simulink model "TrajectoryTracking_2015b_000"  (R2017a)
settings: Solver=ode45  StartTime=0.0  StopTime=125  RelTol=1e-3
values from neighbouring files (symbols this model uses):
  tau_d_1 = C_RB1+C_A1+D1+G1    [DesiredInputOptimalConfiguration.m]
  tau_d_2 = C_RB2+C_A2+D2+G2    [DesiredInputOptimalConfiguration.m]
  tau_d_3 = C_RB3+C_A3+D3+G3    [DesiredInputOptimalConfiguration.m]
  tau_d_4 = C_RB4+C_A4+D4+G4    [DesiredInputOptimalConfiguration.m]
  tau_d_5 = C_RB5+C_A5+D5+G5    [DesiredInputOptimalConfiguration.m]
  tau_d_6 = C_RB6+C_A6+D6+G6    [DesiredInputOptimalConfiguration.m]
  tau_d_7 = C_RB7+C_A7+D7+G7    [DesiredInputOptimalConfiguration.m]
undefined symbols (not defined in the file or in its folder): angular_velocity_pitch_1, angular_velocity_pitch_2, angular_velocity_roll_1, angular_velocity_roll_2, angular_velocity_yaw_1, angular_velocity_yaw_2, B_input, d_H, K1, K2, linear_velocity_x_1, linear_velocity_x_2, linear_velocity_y_1, linear_velocity_y_2, linear_velocity_z_1, linear_velocity_z_2, pitch_angle_1, pitch_angle_2, roll_angle_1, roll_angle_2, t_1_last, t_e_1, t_e_2, u_d_1, u_d_2, u_d_optimized, veh, x1, x2, y1, y2, yaw_angle_1, yaw_angle_2, z1, z2
undefined symbols (not defined in the file): a_F1, a_F2, a_F3, a_F4, b_F1, b_F2, b_F3, b_F4, b_T1_optimized, b_T2_optimized, d_T1_optimized, d_T2_optimized, gamma_F1_optimized, gamma_F2_optimized, gamma_F3_optimized, gamma_F4_optimized, r_T1_optimized, r_T2_optimized, x_F1_optimized, x_F2_optimized, x_F3_optimized, x_F4_optimized
libraries: sharedtransform x1, shared6dofsys x1
(part 1 of 2)
settings Model: Creator=yongyu  LastModifiedBy=yongyu
settings OptimizationCC: LifeSpan=inf
settings DebuggingCC: SFExecutionAtInitializationDiag=none
settings HardwareCC: ProdBitPerSizeT=32  ProdBitPerPtrDiffT=32  ProdWordSize=32  ProdHWDeviceType=Specified

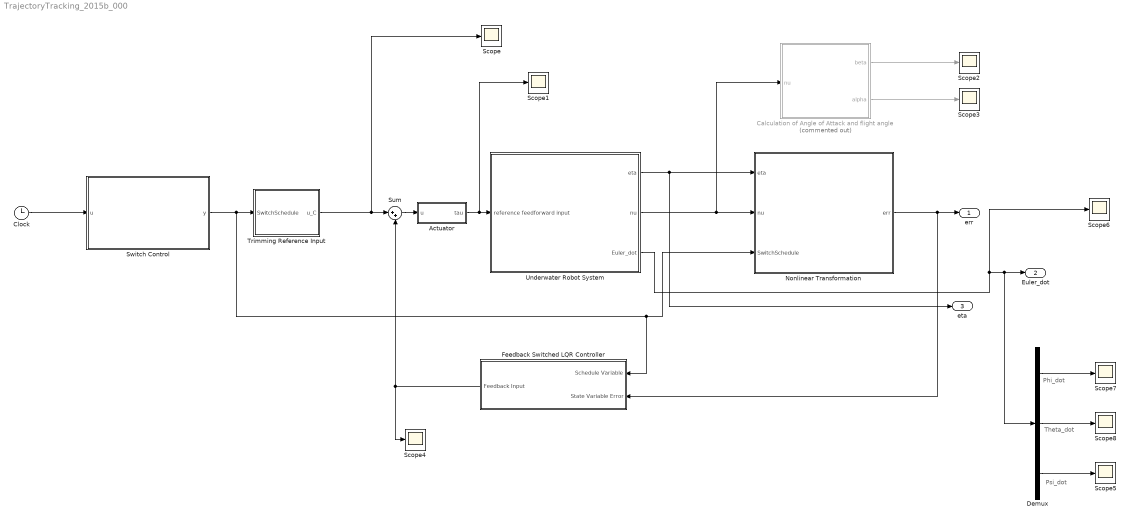
== system TrajectoryTracking_2015b_000 ==
  note: Theta_dot
  note: Phi_dot
  note: Psi_dot
  Actuator : Subsystem
  Calculation of Angle of Attack and flight angle : Subsystem  Commented=on
  Clock : Clock
  Demux : Demux  Outputs=3
  Feedback Switched LQR Controller : Subsystem
  Nonlinear Transformation : Subsystem
  Scope{,1..8} (9 alike) : Scope
  Sum : Sum  Inputs=|++
  Switch Control : MATLAB Function  TreatAsAtomicUnit=on
  "Trimming Reference Input " : Subsystem
  Underwater Robot System : Subsystem
  err : Outport
  Euler_dot : Outport  Port=2
  eta : Outport  Port=3
  wires:
  Nonlinear Transformation/1(err) -> err/1, Feedback Switched LQR Controller/2(State Variable Error)
  Calculation of Angle of Attack and flight angle/2(alpha) -> Scope3/1
  Calculation of Angle of Attack and flight angle/1(beta) -> Scope2/1
  "Trimming Reference Input "/1(u_C) -> Scope/1, Sum/1
  Underwater Robot System/1(eta) -> eta/1, Nonlinear Transformation/1(eta)
  Underwater Robot System/2(nu) -> Calculation of Angle of Attack and flight angle/1(nu), Nonlinear Transformation/2(nu)
  Underwater Robot System/3(Euler_dot) -> Scope6/1, Demux/1, Euler_dot/1
  Clock/1 -> Switch Control/1(u)
  Demux/3 -> Scope5/1
  Switch Control/1(y) -> Feedback Switched LQR Controller/1(Schedule Variable), Nonlinear Transformation/3(SwitchSchedule), "Trimming Reference Input "/1(SwitchSchedule)
  Demux/1 -> Scope7/1
  Demux/2 -> Scope8/1
  Sum/1 -> Actuator/1(u)
  Actuator/1(tau) -> Scope1/1, Underwater Robot System/1("reference feedforward input ")
  Feedback Switched LQR Controller/1(Feedback Input) -> Sum/2, Scope4/1

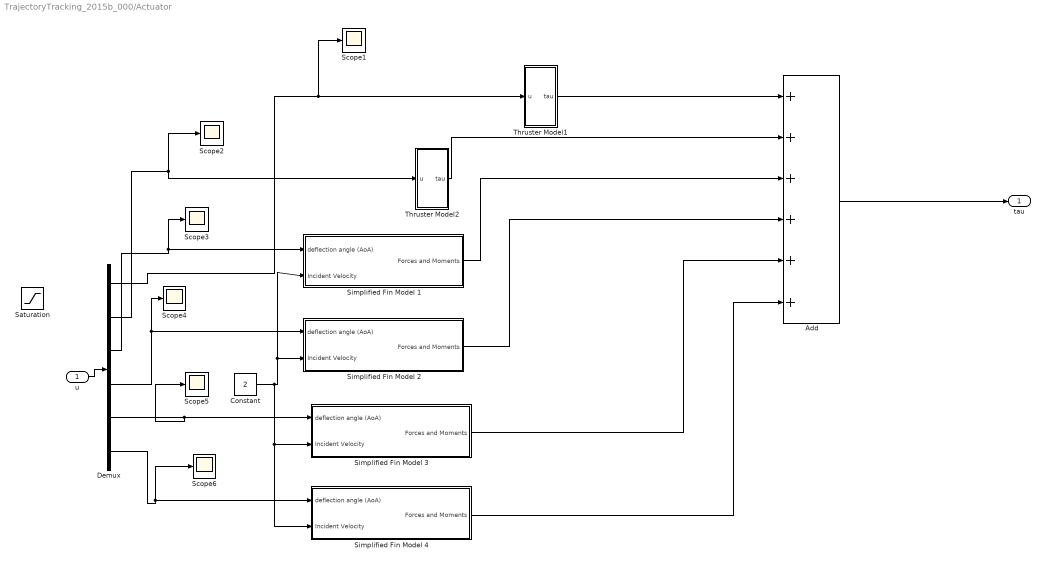
== system TrajectoryTracking_2015b_000/Actuator ==
  u : Inport
  Add : Sum  Inputs=++++++
  Constant : Constant  Value=2
  Demux : Demux  Outputs=6
  Saturation : Saturate  UpperLimit=[40 40 40 40 40 40]  LowerLimit=[-35 -35 -35 -35 -35 -35]
  Scope{1..6} (6 alike) : Scope
  "Simplified Fin Model 1 " : Subsystem  mask{x_F=x_F1_optimized, gama_F=gamma_F1_optimized, a_F=a_F1, b_F=b_F1, C_L=0.3, C_D=0, d_H=d_H, rho=1033}
      mask prompts: x_F "Position of fin middle in body frame {b} in cylinderic coordinate"; gama_F "Rotation angle of the fin (radian)"; a_F "Length of the fin (m)"; b_F "Width of the fin (m)"; C_L "Lift coefficient"; C_D "Drag coefficient"; d_H "Diameter of hull cylinder (m)"; rho "Fluid density"
      mask DialogControl DescTextVar Prompt: Simplified Model for fin (under assumption of small angle of attack)
  Simplified Fin Model 2 : Subsystem  mask{x_F=x_F2_optimized, gama_F=gamma_F2_optimized, a_F=a_F2, b_F=b_F2, C_L=0.3, C_D=0, d_H=d_H, rho=1033}
      mask prompts: x_F "Position of fin middle in body frame {b} in cylinderic coordinate"; gama_F "Rotation angle of the fin (radian)"; a_F "Length of the fin (m)"; b_F "Width of the fin (m)"; C_L "Lift coefficient"; C_D "Drag coefficient"; d_H "Diameter of hull cylinder (m)"; rho "Fluid density"
      mask DialogControl DescTextVar Prompt: Simplified Model for fin (under assumption of small angle of attack)
  Simplified Fin Model 3 : Subsystem  mask{x_F=x_F3_optimized, gama_F=gamma_F3_optimized, a_F=a_F3, b_F=b_F3, C_L=0.3, C_D=0, d_H=d_H, rho=1033}
      mask prompts: x_F "Position of fin middle in body frame {b} in cylinderic coordinate"; gama_F "Rotation angle of the fin (radian)"; a_F "Length of the fin (m)"; b_F "Width of the fin (m)"; C_L "Lift coefficient"; C_D "Drag coefficient"; d_H "Diameter of hull cylinder (m)"; rho "Fluid density"
      mask DialogControl DescTextVar Prompt: Simplified Model for fin (under assumption of small angle of attack)
  Simplified Fin Model 4 : Subsystem  mask{x_F=x_F4_optimized, gama_F=gamma_F4_optimized, a_F=a_F4, b_F=b_F4, C_L=0.3, C_D=0, d_H=d_H, rho=1033}
      mask prompts: x_F "Position of fin middle in body frame {b} in cylinderic coordinate"; gama_F "Rotation angle of the fin (radian)"; a_F "Length of the fin (m)"; b_F "Width of the fin (m)"; C_L "Lift coefficient"; C_D "Drag coefficient"; d_H "Diameter of hull cylinder (m)"; rho "Fluid density"
      mask DialogControl DescTextVar Prompt: Simplified Model for fin (under assumption of small angle of attack)
  Thruster Model1 : Subsystem  mask{d_T=d_T1_optimized, b_T=b_T1_optimized, r_T=r_T1_optimized, lambda_T=veh.lambda1}
      mask DialogControl DescTextVar Prompt: Model of Thruster
  Thruster Model2 : Subsystem  mask{d_T=d_T2_optimized, b_T=b_T2_optimized, r_T=r_T2_optimized, lambda_T=veh.lambda2}
      mask DialogControl DescTextVar Prompt: Model of Thruster
  tau : Outport
  wires:
  Simplified Fin Model 3/1(Forces and Moments) -> Add/5
  "Simplified Fin Model 1 "/1(Forces and Moments) -> Add/3
  Simplified Fin Model 2/1(Forces and Moments) -> Add/4
  Thruster Model2/1(tau) -> Add/2
  Simplified Fin Model 4/1(Forces and Moments) -> Add/6
  Add/1 -> tau/1
  Thruster Model1/1(tau) -> Add/1
  Demux/1 -> Thruster Model1/1(u), Scope1/1
  Demux/2 -> Thruster Model2/1(u), Scope2/1
  Demux/3 -> "Simplified Fin Model 1 "/1(deflection angle (AoA)), Scope3/1
  Demux/4 -> Scope4/1, Simplified Fin Model 2/1(deflection angle (AoA))
  Demux/5 -> Scope5/1, Simplified Fin Model 3/1(deflection angle (AoA))
  Demux/6 -> Simplified Fin Model 4/1(deflection angle (AoA)), Scope6/1
  u/1 -> Demux/1
  Constant/1 -> Simplified Fin Model 4/2(Incident Velocity), Simplified Fin Model 3/2(Incident Velocity), Simplified Fin Model 2/2(Incident Velocity), "Simplified Fin Model 1 "/2(Incident Velocity)

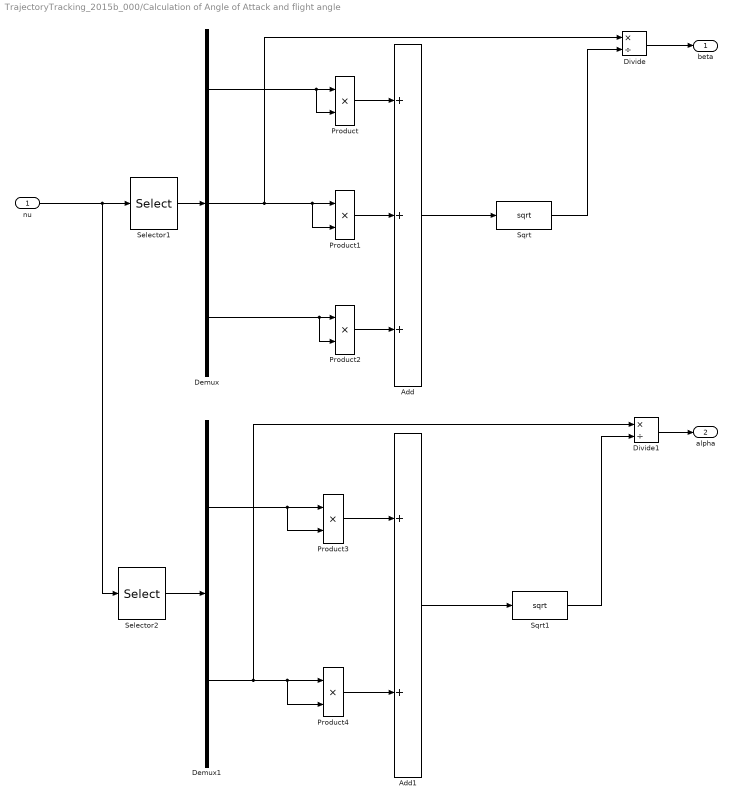
== system TrajectoryTracking_2015b_000/Calculation of Angle of Attack and flight angle ==
  nu : Inport
  Add : Sum  Inputs=+++
  Add1 : Sum
  Demux : Demux  Outputs=3
  Demux1 : Demux  Outputs=2
  Divide : Product  Inputs=*/
  Divide1 : Product  Inputs=*/
  Product{,1..4} (5 alike) : Product
  Selector1 : Selector  InputPortWidth=6  IndexOptions=Index vector (dialog)  Indices=[1 2 3]  OutputSizes=1
  Selector2 : Selector  InputPortWidth=6  IndexOptions=Index vector (dialog)  Indices=[1 3]  OutputSizes=1
  Sqrt : Sqrt  SaturateOnIntegerOverflow=on
  Sqrt1 : Sqrt  SaturateOnIntegerOverflow=on
  beta : Outport
  alpha : Outport  Port=2
  wires:
  nu/1 -> Selector2/1, Selector1/1
  Selector1/1 -> Demux/1
  Demux/1 -> Product/2, Product/1
  Demux/2 -> Product1/2, Product1/1, Divide/1
  Demux/3 -> Product2/2, Product2/1
  Product/1 -> Add/1
  Product1/1 -> Add/2
  Product2/1 -> Add/3
  Add/1 -> Sqrt/1
  Sqrt/1 -> Divide/2
  Divide/1 -> beta/1
  Selector2/1 -> Demux1/1
  Demux1/1 -> Product3/2, Product3/1
  Demux1/2 -> Divide1/1, Product4/2, Product4/1
  Product3/1 -> Add1/1
  Product4/1 -> Add1/2
  Add1/1 -> Sqrt1/1
  Sqrt1/1 -> Divide1/2
  Divide1/1 -> alpha/1

== system TrajectoryTracking_2015b_000/Feedback Switched LQR Controller ==
  Schedule Variable : Inport
  State Variable Error : Inport  Port=2
  Constant1 : Constant  Value=-K2
  Constant7 : Constant  Value=-K1
  Multiport Switch : MultiPortSwitch  Inputs=2
  Product : Product  Multiplication=Matrix(*)
  Feedback Input : Outport
  wires:
  Constant7/1 -> Multiport Switch/2
  Constant1/1 -> Multiport Switch/3
  Multiport Switch/1 -> Product/1
  Product/1 -> Feedback Input/1
  State Variable Error/1 -> Product/2
  Schedule Variable/1 -> Multiport Switch/1

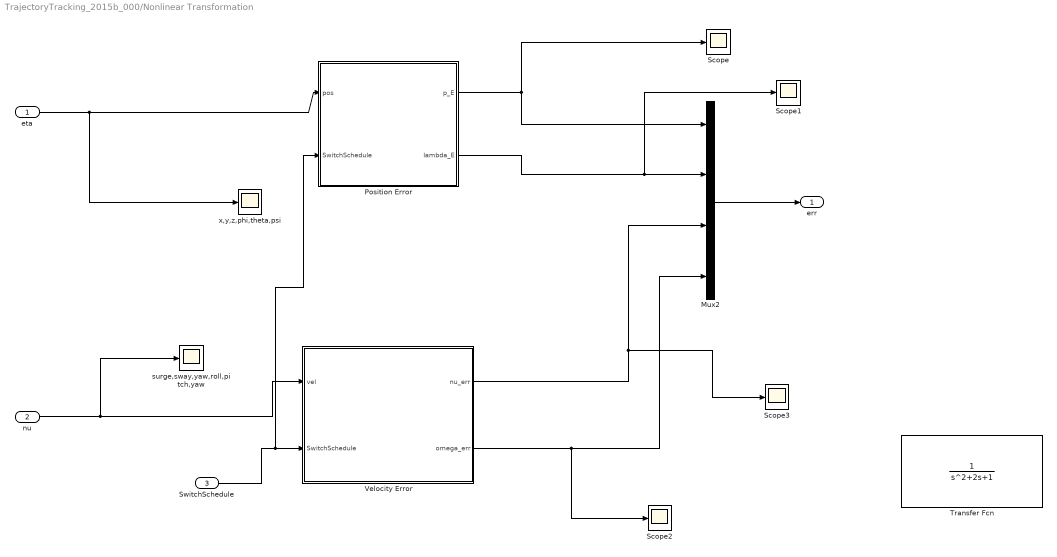
== system TrajectoryTracking_2015b_000/Nonlinear Transformation ==
  eta : Inport
  nu : Inport  Port=2
  SwitchSchedule : Inport  Port=3
  Mux2 : Mux
  "Position Error " : Subsystem
  Scope{,1..3} (4 alike) : Scope
  Transfer Fcn : TransferFcn
  "Velocity Error " : Subsystem
  surge,sway,yaw,roll,pitch,yaw : Scope
  x,y,z,phi,theta,psi : Scope
  err : Outport
  wires:
  nu/1 -> surge,sway,yaw,roll,pitch,yaw/1, "Velocity Error "/1(vel)
  eta/1 -> x,y,z,phi,theta,psi/1, "Position Error "/1(pos)
  Mux2/1 -> err/1
  "Position Error "/1(p_E) -> Scope/1, Mux2/1
  "Position Error "/2(lambda_E) -> Scope1/1, Mux2/2
  "Velocity Error "/1(nu_err) -> Scope3/1, Mux2/3
  "Velocity Error "/2(omega_err) -> Scope2/1, Mux2/4
  SwitchSchedule/1 -> "Position Error "/2(SwitchSchedule), "Velocity Error "/2(SwitchSchedule)

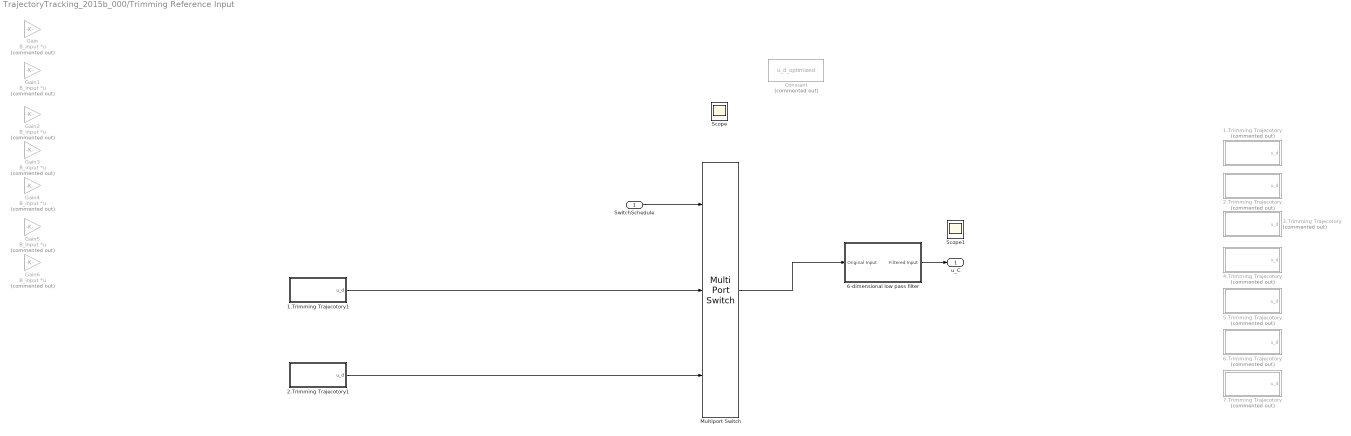
== system TrajectoryTracking_2015b_000/Trimming Reference Input  ==
  SwitchSchedule : Inport
  1.Trimming Trajecotory : Subsystem  Commented=on
  1.Trimming Trajecotory1 : Subsystem
  2.Trimming Trajecotory : Subsystem  Commented=on
  2.Trimming Trajecotory1 : Subsystem
  3.Trimming Trajecotory : Subsystem  Commented=on
  4.Trimming Trajecotory : Subsystem  Commented=on
  5.Trimming Trajecotory : Subsystem  Commented=on
  6-dimensional low pass filter : Subsystem
  6.Trimming Trajecotory : Subsystem  Commented=on
  7.Trimming Trajecotory : Subsystem  Commented=on
  Constant : Constant  Commented=on  Value=u_d_optimized
  Gain{,1..6} (7 alike) : Gain  Commented=on  Gain=B_input  Multiplication=Matrix(K*u)
  Multiport Switch : MultiPortSwitch  Inputs=2
  Scope : Scope
  Scope1 : Scope
  u_C : Outport
  wires:
  SwitchSchedule/1 -> Multiport Switch/1
  1.Trimming Trajecotory1/1(u_d) -> Multiport Switch/2
  6-dimensional low pass filter/1(Filtered Input) -> u_C/1
  Multiport Switch/1 -> 6-dimensional low pass filter/1(Original Input)
  2.Trimming Trajecotory1/1(u_d) -> Multiport Switch/3

== system TrajectoryTracking_2015b_000/Underwater Robot System ==
  "reference feedforward input " : Inport
  Demux : Demux  Outputs=6
  Underwater Robot System : Subsystem
  eta : Outport
  nu : Outport  Port=2
  Euler_dot : Outport  Port=3
  wires:
  Underwater Robot System/1(eta) -> eta/1
  Underwater Robot System/2(nu) -> nu/1
  Demux/6 -> Underwater Robot System/6(N)
  Demux/5 -> Underwater Robot System/5(M)
  Demux/4 -> Underwater Robot System/4(K)
  Demux/3 -> Underwater Robot System/3(Z)
  Demux/2 -> Underwater Robot System/2(Y)
  Demux/1 -> Underwater Robot System/1(X)
  "reference feedforward input "/1 -> Demux/1
  Underwater Robot System/3(Euler_dot) -> Euler_dot/1

== system TrajectoryTracking_2015b_000/Actuator/Simplified Fin Model 1  ==
  deflection angle (AoA) : Inport
  Incident Velocity : Inport  Port=2
  Drag Forces and Moments : Subsystem
  Lift Forces and Moments : Subsystem
  Sum : Sum  Inputs=|++
  Forces and Moments : Outport
  wires:
  deflection angle (AoA)/1 -> Drag Forces and Moments/1(AoA), Lift Forces and Moments/1(AoA)
  Incident Velocity/1 -> Drag Forces and Moments/2(u), Lift Forces and Moments/2(u)
  Lift Forces and Moments/1("F_L, m_L") -> Sum/1
  Sum/1 -> Forces and Moments/1
  Drag Forces and Moments/1(F_D,m_D) -> Sum/2

== system TrajectoryTracking_2015b_000/Actuator/Simplified Fin Model 2 ==
  deflection angle (AoA) : Inport
  Incident Velocity : Inport  Port=2
  Drag Forces and Moments : Subsystem
  Lift Forces and Moments : Subsystem
  Sum : Sum  Inputs=|++
  Forces and Moments : Outport
  wires:
  deflection angle (AoA)/1 -> Drag Forces and Moments/1(AoA), Lift Forces and Moments/1(AoA)
  Incident Velocity/1 -> Drag Forces and Moments/2(u), Lift Forces and Moments/2(u)
  Lift Forces and Moments/1("F_L, m_L") -> Sum/1
  Sum/1 -> Forces and Moments/1
  Drag Forces and Moments/1(F_D,m_D) -> Sum/2

== system TrajectoryTracking_2015b_000/Actuator/Simplified Fin Model 3 ==
  deflection angle (AoA) : Inport
  Incident Velocity : Inport  Port=2
  Drag Forces and Moments : Subsystem
  Lift Forces and Moments : Subsystem
  Sum : Sum  Inputs=|++
  Forces and Moments : Outport
  wires:
  deflection angle (AoA)/1 -> Drag Forces and Moments/1(AoA), Lift Forces and Moments/1(AoA)
  Incident Velocity/1 -> Drag Forces and Moments/2(u), Lift Forces and Moments/2(u)
  Lift Forces and Moments/1("F_L, m_L") -> Sum/1
  Sum/1 -> Forces and Moments/1
  Drag Forces and Moments/1(F_D,m_D) -> Sum/2

== system TrajectoryTracking_2015b_000/Actuator/Simplified Fin Model 4 ==
  deflection angle (AoA) : Inport
  Incident Velocity : Inport  Port=2
  Drag Forces and Moments : Subsystem
  Lift Forces and Moments : Subsystem
  Sum : Sum  Inputs=|++
  Forces and Moments : Outport
  wires:
  deflection angle (AoA)/1 -> Drag Forces and Moments/1(AoA), Lift Forces and Moments/1(AoA)
  Incident Velocity/1 -> Drag Forces and Moments/2(u), Lift Forces and Moments/2(u)
  Lift Forces and Moments/1("F_L, m_L") -> Sum/1
  Drag Forces and Moments/1(F_D,m_D) -> Sum/2
  Sum/1 -> Forces and Moments/1

== system TrajectoryTracking_2015b_000/Actuator/Thruster Model1 ==
  u : Inport
  3x3 cross product : Subsystem
  Constant : Constant  Value=r_T
  Constant1 : Constant  Value=d_T
  Display : Display
  Gain : Gain  Gain=d_T  Multiplication=Matrix(K*u)
  Gain1 : Gain  Gain=b_T*lambda_T*d_T  Multiplication=Matrix(K*u)
  Mux : Mux  Inputs=2
  Product : Product
  Sum : Sum  Inputs=|++
  tau : Outport
  wires:
  u/1 -> Product/1, Gain1/1, Gain/1
  Constant/1 -> 3x3 cross product/1(a)
  Constant1/1 -> 3x3 cross product/2(b)
  Gain1/1 -> Sum/1
  3x3 cross product/1(c) -> Product/2
  Gain/1 -> Mux/1
  Mux/1 -> tau/1
  Sum/1 -> Mux/2
  Product/1 -> Sum/2, Display/1

== system TrajectoryTracking_2015b_000/Actuator/Thruster Model2 ==
  u : Inport
  3x3 cross product : Subsystem
  Constant : Constant  Value=r_T
  Constant1 : Constant  Value=d_T
  Display : Display
  Gain : Gain  Gain=d_T  Multiplication=Matrix(K*u)
  Gain1 : Gain  Gain=b_T*lambda_T*d_T  Multiplication=Matrix(K*u)
  Mux : Mux  Inputs=2
  Product : Product
  Sum : Sum  Inputs=|++
  tau : Outport
  wires:
  u/1 -> Product/1, Gain1/1, Gain/1
  Constant/1 -> 3x3 cross product/1(a)
  Constant1/1 -> 3x3 cross product/2(b)
  Gain1/1 -> Sum/1
  3x3 cross product/1(c) -> Product/2
  Gain/1 -> Mux/1
  Mux/1 -> tau/1
  Sum/1 -> Mux/2
  Product/1 -> Sum/2, Display/1

== system TrajectoryTracking_2015b_000/Nonlinear Transformation/Position Error  ==
  pos : Inport
  SwitchSchedule : Inport  Port=2
  Nonlinear Orientation Transformation : Subsystem
  Nonlinear Position Transformation : Subsystem
  Selector1 : Selector  InputPortWidth=6  IndexOptions=Index vector (dialog)  Indices=[1 2 3]  OutputSizes=1
  Selector2 : Selector  InputPortWidth=6  IndexOptions=Index vector (dialog)  Indices=[4 5 6]  OutputSizes=1
  p_E : Outport
  lambda_E : Outport  Port=2
  wires:
  pos/1 -> Selector2/1, Selector1/1
  Selector2/1 -> Nonlinear Position Transformation/2(theta), Nonlinear Orientation Transformation/1(theta)
  Selector1/1 -> Nonlinear Position Transformation/1(x,y,z)
  Nonlinear Position Transformation/1(p_E) -> p_E/1
  Nonlinear Orientation Transformation/1(lambda_E) -> lambda_E/1
  SwitchSchedule/1 -> Nonlinear Orientation Transformation/2(SwitchSchedule), Nonlinear Position Transformation/3(SwitchSchedule)

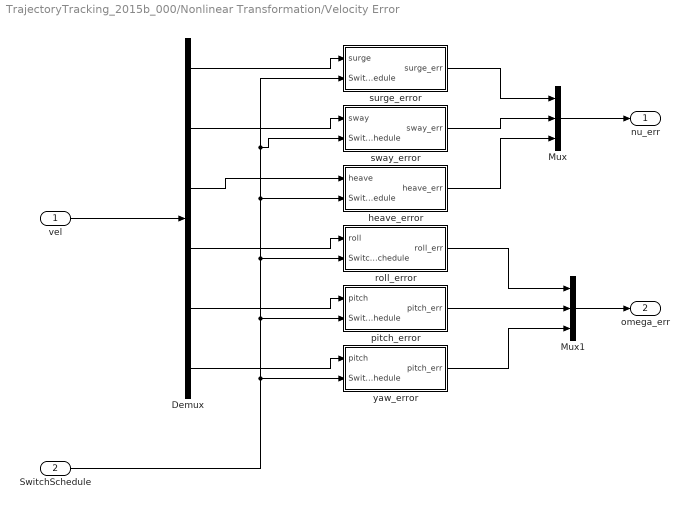
== system TrajectoryTracking_2015b_000/Nonlinear Transformation/Velocity Error  ==
  vel : Inport
  SwitchSchedule : Inport  Port=2
  Demux : Demux  Outputs=6
  Mux : Mux  Inputs=3
  Mux1 : Mux  Inputs=3
  heave_error : Subsystem
  pitch_error : Subsystem
  roll_error : Subsystem
  surge_error : Subsystem
  sway_error : Subsystem
  yaw_error : Subsystem
  nu_err : Outport
  omega_err : Outport  Port=2
  wires:
  vel/1 -> Demux/1
  Mux/1 -> nu_err/1
  Demux/1 -> surge_error/1(surge)
  Demux/2 -> sway_error/1(sway)
  Demux/3 -> heave_error/1(heave)
  Demux/4 -> roll_error/1(roll)
  Demux/5 -> pitch_error/1(pitch)
  Demux/6 -> yaw_error/1(pitch)
  surge_error/1(surge_err) -> Mux/1
  sway_error/1(sway_err) -> Mux/2
  heave_error/1(heave_err) -> Mux/3
  roll_error/1(roll_err) -> Mux1/1
  pitch_error/1(pitch_err) -> Mux1/2
  yaw_error/1(pitch_err) -> Mux1/3
  Mux1/1 -> omega_err/1
  SwitchSchedule/1 -> yaw_error/2(SwitchSchedule), pitch_error/2(SwitchSchedule), roll_error/2(SwitchSchedule), sway_error/2(SwitchSchedule), surge_error/2(SwitchSchedule), heave_error/2(SwitchSchedule)

== system TrajectoryTracking_2015b_000/Trimming Reference Input /1.Trimming Trajecotory ==
  Constant : Constant  Value=tau_d_1(1,1,1)
  Constant1 : Constant  Value=tau_d_1(2,1,1)
  Constant2 : Constant  Value=tau_d_1(3,1,1)
  Constant3 : Constant  Value=tau_d_1(4,1,1)
  Constant4 : Constant  Value=tau_d_1(5,1,1)
  Constant5 : Constant  Value=tau_d_1(6,1,1)
  Mux : Mux  Inputs=6
  u_d : Outport
  wires:
  Mux/1 -> u_d/1
  Constant/1 -> Mux/1
  Constant1/1 -> Mux/2
  Constant2/1 -> Mux/3
  Constant3/1 -> Mux/4
  Constant4/1 -> Mux/5
  Constant5/1 -> Mux/6

== system TrajectoryTracking_2015b_000/Trimming Reference Input /1.Trimming Trajecotory1 ==
  Constant : Constant  Value=u_d_1
  u_d : Outport
  wires:
  Constant/1 -> u_d/1

== system TrajectoryTracking_2015b_000/Trimming Reference Input /2.Trimming Trajecotory ==
  Constant : Constant  Value=tau_d_2(1,1,1)
  Constant1 : Constant  Value=tau_d_2(2,1,1)
  Constant2 : Constant  Value=tau_d_2(3,1,1)
  Constant3 : Constant  Value=tau_d_2(4,1,1)
  Constant4 : Constant  Value=tau_d_2(5,1,1)
  Constant5 : Constant  Value=tau_d_2(6,1,1)
  Mux : Mux  Inputs=6
  u_d : Outport
  wires:
  Constant4/1 -> Mux/5
  Constant3/1 -> Mux/4
  Constant5/1 -> Mux/6
  Constant2/1 -> Mux/3
  Constant/1 -> Mux/1
  Mux/1 -> u_d/1
  Constant1/1 -> Mux/2

== system TrajectoryTracking_2015b_000/Trimming Reference Input /2.Trimming Trajecotory1 ==
  Constant : Constant  Value=u_d_2
  u_d : Outport
  wires:
  Constant/1 -> u_d/1

== system TrajectoryTracking_2015b_000/Trimming Reference Input /3.Trimming Trajecotory ==
  Constant : Constant  Value=tau_d_3(1,1,1)
  Constant1 : Constant  Value=tau_d_3(2,1,1)
  Constant2 : Constant  Value=tau_d_3(3,1,1)
  Constant3 : Constant  Value=tau_d_3(4,1,1)
  Constant4 : Constant  Value=tau_d_3(5,1,1)
  Constant5 : Constant  Value=tau_d_3(6,1,1)
  Mux : Mux  Inputs=6
  u_d : Outport
  wires:
  Constant3/1 -> Mux/4
  Mux/1 -> u_d/1
  Constant5/1 -> Mux/6
  Constant2/1 -> Mux/3
  Constant4/1 -> Mux/5
  Constant/1 -> Mux/1
  Constant1/1 -> Mux/2

== system TrajectoryTracking_2015b_000/Trimming Reference Input /4.Trimming Trajecotory ==
  Constant : Constant  Value=tau_d_4(1,1,1)
  Constant1 : Constant  Value=tau_d_4(2,1,1)
  Constant2 : Constant  Value=tau_d_4(3,1,1)
  Constant3 : Constant  Value=tau_d_4(4,1,1)
  Constant4 : Constant  Value=tau_d_4(5,1,1)
  Constant5 : Constant  Value=tau_d_4(6,1,1)
  Mux : Mux  Inputs=6
  u_d : Outport
  wires:
  Constant1/1 -> Mux/2
  Constant/1 -> Mux/1
  Constant4/1 -> Mux/5
  Constant2/1 -> Mux/3
  Constant5/1 -> Mux/6
  Mux/1 -> u_d/1
  Constant3/1 -> Mux/4

== system TrajectoryTracking_2015b_000/Trimming Reference Input /5.Trimming Trajecotory ==
  Constant : Constant  Value=tau_d_5(1,1,1)
  Constant1 : Constant  Value=tau_d_5(2,1,1)
  Constant2 : Constant  Value=tau_d_5(3,1,1)
  Constant3 : Constant  Value=tau_d_5(4,1,1)
  Constant4 : Constant  Value=tau_d_5(5,1,1)
  Constant5 : Constant  Value=tau_d_5(6,1,1)
  Mux : Mux  Inputs=6
  u_d : Outport
  wires:
  Constant1/1 -> Mux/2
  Constant/1 -> Mux/1
  Constant4/1 -> Mux/5
  Constant2/1 -> Mux/3
  Constant5/1 -> Mux/6
  Mux/1 -> u_d/1
  Constant3/1 -> Mux/4

== system TrajectoryTracking_2015b_000/Trimming Reference Input /6-dimensional low pass filter ==
  Original Input : Inport
  Demux : Demux  Outputs=6
  Mux : Mux  Inputs=6
  Transfer Fcn{,1..5} (6 alike) : TransferFcn  Denominator=[1 1]
  Filtered Input : Outport
  wires:
  Transfer Fcn/1 -> Mux/1
  Demux/5 -> Transfer Fcn4/1
  Demux/2 -> Transfer Fcn1/1
  Transfer Fcn3/1 -> Mux/4
  Demux/4 -> Transfer Fcn3/1
  Demux/3 -> Transfer Fcn2/1
  Transfer Fcn4/1 -> Mux/5
  Transfer Fcn5/1 -> Mux/6
  Demux/1 -> Transfer Fcn/1
  Transfer Fcn1/1 -> Mux/2
  Transfer Fcn2/1 -> Mux/3
  Demux/6 -> Transfer Fcn5/1
  Mux/1 -> Filtered Input/1
  Original Input/1 -> Demux/1

== system TrajectoryTracking_2015b_000/Trimming Reference Input /6.Trimming Trajecotory ==
  Constant : Constant  Value=tau_d_6(1,1,1)
  Constant1 : Constant  Value=tau_d_6(2,1,1)
  Constant2 : Constant  Value=tau_d_6(3,1,1)
  Constant3 : Constant  Value=tau_d_6(4,1,1)
  Constant4 : Constant  Value=tau_d_6(5,1,1)
  Constant5 : Constant  Value=tau_d_6(6,1,1)
  Mux : Mux  Inputs=6
  u_d : Outport
  wires:
  Constant1/1 -> Mux/2
  Constant/1 -> Mux/1
  Constant4/1 -> Mux/5
  Constant2/1 -> Mux/3
  Constant5/1 -> Mux/6
  Mux/1 -> u_d/1
  Constant3/1 -> Mux/4

== system TrajectoryTracking_2015b_000/Trimming Reference Input /7.Trimming Trajecotory ==
  Constant : Constant  Value=tau_d_7(1,1,1)
  Constant1 : Constant  Value=tau_d_7(2,1,1)
  Constant2 : Constant  Value=tau_d_7(3,1,1)
  Constant3 : Constant  Value=tau_d_7(4,1,1)
  Constant4 : Constant  Value=tau_d_7(5,1,1)
  Constant5 : Constant  Value=tau_d_7(6,1,1)
  Mux : Mux  Inputs=6
  u_d : Outport
  wires:
  Constant1/1 -> Mux/2
  Constant/1 -> Mux/1
  Constant4/1 -> Mux/5
  Constant2/1 -> Mux/3
  Constant5/1 -> Mux/6
  Mux/1 -> u_d/1
  Constant3/1 -> Mux/4

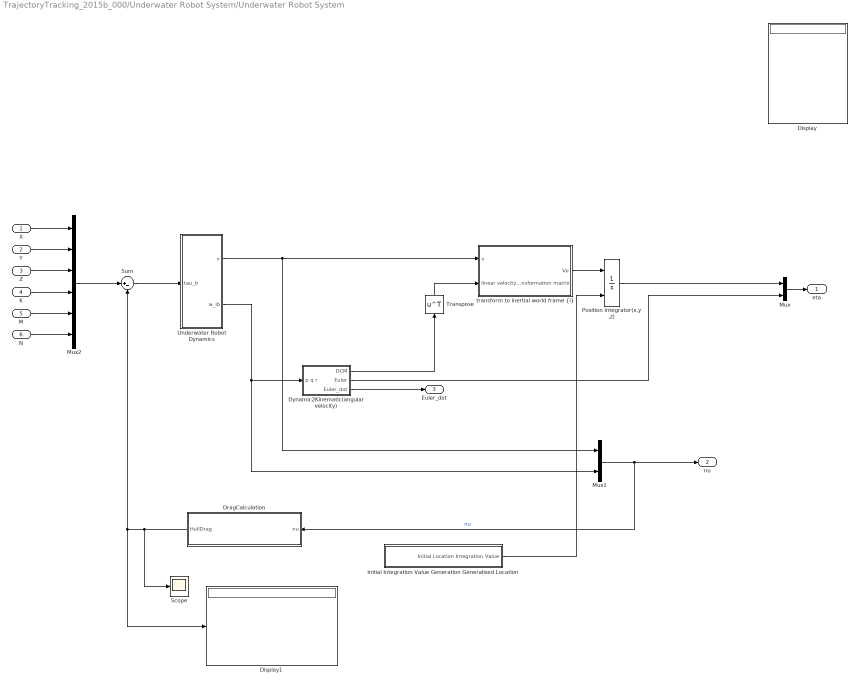
== system TrajectoryTracking_2015b_000/Underwater Robot System/Underwater Robot System ==
  X : Inport
  Y : Inport  Port=2
  Z : Inport  Port=3
  K : Inport  Port=4
  M : Inport  Port=5
  N : Inport  Port=6
  Display : Display
  Display1 : Display
  DragCalculation : Subsystem
  Dynamic2Kinematic(angular velocity) : Subsystem
  Initial Integration Value Generation Generalised Location : Subsystem
  Mux : Mux  Inputs=2
  Mux1 : Mux  Inputs=2
  Mux2 : Mux  Inputs=6
  Position Integrator(x,y,z) : Integrator  InitialConditionSource=external
  Scope : Scope
  Sum : Sum  Inputs=|+-
  Transpose : Math  Operator=transpose  SaturateOnIntegerOverflow=on
  "Underwater Robot Dynamics " : Subsystem
  "transform to inertial world frame {i}" : Subsystem
  eta : Outport
  nu : Outport  Port=2
  Euler_dot : Outport  Port=3
  wires:
  Transpose/1 -> "transform to inertial world frame {i}"/2(linear velocity transformation matrix)
  Mux1/1 -> nu/1, DragCalculation/1(nu)  "nu"
  Mux/1 -> eta/1
  "transform to inertial world frame {i}"/1(Ve) -> Position Integrator(x,y,z)/1
  Position Integrator(x,y,z)/1 -> Mux/1
  "Underwater Robot Dynamics "/2(w_ib) -> Mux1/2, Dynamic2Kinematic(angular velocity)/1("p q r ")
  "Underwater Robot Dynamics "/1(v) -> Mux1/1, "transform to inertial world frame {i}"/1(v)
  N/1 -> Mux2/6
  M/1 -> Mux2/5
  K/1 -> Mux2/4
  Z/1 -> Mux2/3
  Y/1 -> Mux2/2
  X/1 -> Mux2/1
  Dynamic2Kinematic(angular velocity)/1(DCM) -> Transpose/1
  Dynamic2Kinematic(angular velocity)/2(Euler) -> Mux/2
  Initial Integration Value Generation Generalised Location/1(Initial Location Integration Value) -> Position Integrator(x,y,z)/2
  Dynamic2Kinematic(angular velocity)/3(Euler_dot) -> Euler_dot/1
  DragCalculation/1(HullDrag) -> Scope/1, Display1/1, Sum/2
  Mux2/1 -> Sum/1
  Sum/1 -> "Underwater Robot Dynamics "/1(tau_b)

== system TrajectoryTracking_2015b_000/Actuator/Simplified Fin Model 1 /Drag Forces and Moments ==
  AoA : Inport
  u : Inport  Port=2
  "Drag Force " : Subsystem
  Geometric Center of fin : Subsystem
  Mux : Mux  Inputs=2
  Product1 : Product  Multiplication=Matrix(*)
  F_D,m_D : Outport
  wires:
  Geometric Center of fin/1(r_F) -> Product1/1
  "Drag Force "/1(Drag Force) -> Mux/1, Product1/2
  u/1 -> "Drag Force "/2(u)
  AoA/1 -> "Drag Force "/1(AoA)
  Product1/1 -> Mux/2
  Mux/1 -> F_D,m_D/1

== system TrajectoryTracking_2015b_000/Actuator/Simplified Fin Model 1 /Lift Forces and Moments ==
  AoA : Inport
  u : Inport  Port=2
  Geometric Center of fin : Subsystem
  "Lift Force " : Subsystem
  Mux : Mux  Inputs=2
  Product : Product  Multiplication=Matrix(*)
  "F_L, m_L" : Outport
  wires:
  Geometric Center of fin/1(r_F) -> Product/1
  u/1 -> "Lift Force "/1(u)
  AoA/1 -> "Lift Force "/2(AoA)
  "Lift Force "/1(Lift Force) -> Mux/1, Product/2
  Product/1 -> Mux/2
  Mux/1 -> "F_L, m_L"/1

== system TrajectoryTracking_2015b_000/Actuator/Simplified Fin Model 2/Drag Forces and Moments ==
  AoA : Inport
  u : Inport  Port=2
  "Drag Force " : Subsystem
  Geometric Center of fin : Subsystem
  Mux : Mux  Inputs=2
  Product1 : Product  Multiplication=Matrix(*)
  F_D,m_D : Outport
  wires:
  Geometric Center of fin/1(r_F) -> Product1/1
  "Drag Force "/1(Drag Force) -> Mux/1, Product1/2
  Product1/1 -> Mux/2
  u/1 -> "Drag Force "/2(u)
  AoA/1 -> "Drag Force "/1(AoA)
  Mux/1 -> F_D,m_D/1

== system TrajectoryTracking_2015b_000/Actuator/Simplified Fin Model 2/Lift Forces and Moments ==
  AoA : Inport
  u : Inport  Port=2
  Geometric Center of fin : Subsystem
  "Lift Force " : Subsystem
  Mux : Mux  Inputs=2
  Product : Product  Multiplication=Matrix(*)
  "F_L, m_L" : Outport
  wires:
  Geometric Center of fin/1(r_F) -> Product/1
  u/1 -> "Lift Force "/1(u)
  AoA/1 -> "Lift Force "/2(AoA)
  "Lift Force "/1(Lift Force) -> Mux/1, Product/2
  Product/1 -> Mux/2
  Mux/1 -> "F_L, m_L"/1

== system TrajectoryTracking_2015b_000/Actuator/Simplified Fin Model 3/Drag Forces and Moments ==
  AoA : Inport
  u : Inport  Port=2
  "Drag Force " : Subsystem
  Geometric Center of fin : Subsystem
  Mux : Mux  Inputs=2
  Product1 : Product  Multiplication=Matrix(*)
  F_D,m_D : Outport
  wires:
  Geometric Center of fin/1(r_F) -> Product1/1
  "Drag Force "/1(Drag Force) -> Mux/1, Product1/2
  u/1 -> "Drag Force "/2(u)
  AoA/1 -> "Drag Force "/1(AoA)
  Mux/1 -> F_D,m_D/1
  Product1/1 -> Mux/2

== system TrajectoryTracking_2015b_000/Actuator/Simplified Fin Model 3/Lift Forces and Moments ==
  AoA : Inport
  u : Inport  Port=2
  Geometric Center of fin : Subsystem
  "Lift Force " : Subsystem
  Mux : Mux  Inputs=2
  Product : Product  Multiplication=Matrix(*)
  "F_L, m_L" : Outport
  wires:
  Geometric Center of fin/1(r_F) -> Product/1
  u/1 -> "Lift Force "/1(u)
  AoA/1 -> "Lift Force "/2(AoA)
  "Lift Force "/1(Lift Force) -> Mux/1, Product/2
  Product/1 -> Mux/2
  Mux/1 -> "F_L, m_L"/1

== system TrajectoryTracking_2015b_000/Actuator/Simplified Fin Model 4/Drag Forces and Moments ==
  AoA : Inport
  u : Inport  Port=2
  "Drag Force " : Subsystem
  Geometric Center of fin : Subsystem
  Mux : Mux  Inputs=2
  Product1 : Product  Multiplication=Matrix(*)
  F_D,m_D : Outport
  wires:
  Geometric Center of fin/1(r_F) -> Product1/1
  "Drag Force "/1(Drag Force) -> Mux/1, Product1/2
  Product1/1 -> Mux/2
  u/1 -> "Drag Force "/2(u)
  AoA/1 -> "Drag Force "/1(AoA)
  Mux/1 -> F_D,m_D/1

== system TrajectoryTracking_2015b_000/Actuator/Simplified Fin Model 4/Lift Forces and Moments ==
  AoA : Inport
  u : Inport  Port=2
  Geometric Center of fin : Subsystem
  "Lift Force " : Subsystem
  Mux : Mux  Inputs=2
  Product : Product  Multiplication=Matrix(*)
  "F_L, m_L" : Outport
  wires:
  Geometric Center of fin/1(r_F) -> Product/1
  u/1 -> "Lift Force "/1(u)
  AoA/1 -> "Lift Force "/2(AoA)
  "Lift Force "/1(Lift Force) -> Mux/1, Product/2
  Product/1 -> Mux/2
  Mux/1 -> "F_L, m_L"/1

== system TrajectoryTracking_2015b_000/Actuator/Thruster Model1/3x3 cross product ==
  a : Inport
  b : Inport  Port=2
  Product : Product  SaturateOnIntegerOverflow=on  InputSameDT=on  OutDataTypeStr=Inherit: Same as first input
  Product1 : Product  SaturateOnIntegerOverflow=on  InputSameDT=on  OutDataTypeStr=Inherit: Same as first input
  Selector : Selector  InputPortWidth=3  IndexOptions=Index vector (dialog)  Indices=[2 3 1]  OutputSizes=1
  Selector1 : Selector  InputPortWidth=3  IndexOptions=Index vector (dialog)  Indices=[3 1 2]  OutputSizes=1
  Selector2 : Selector  InputPortWidth=3  IndexOptions=Index vector (dialog)  Indices=[2 3 1]  OutputSizes=1
  Selector3 : Selector  InputPortWidth=3  IndexOptions=Index vector (dialog)  Indices=[3 1 2]  OutputSizes=1
  Sum : Sum  Inputs=+|-  SaturateOnIntegerOverflow=on  InputSameDT=on  OutDataTypeStr=Inherit: Same as first input
  c : Outport  InitialOutput=0
  wires:
  Selector3/1 -> Product1/1
  Selector2/1 -> Product1/2
  Product1/1 -> Sum/2
  Selector1/1 -> Product/2
  Product/1 -> Sum/1
  a/1 -> Selector3/1, Selector/1
  Selector/1 -> Product/1
  b/1 -> Selector2/1, Selector1/1
  Sum/1 -> c/1

== system TrajectoryTracking_2015b_000/Actuator/Thruster Model2/3x3 cross product ==
  a : Inport
  b : Inport  Port=2
  Product : Product  SaturateOnIntegerOverflow=on  InputSameDT=on  OutDataTypeStr=Inherit: Same as first input
  Product1 : Product  SaturateOnIntegerOverflow=on  InputSameDT=on  OutDataTypeStr=Inherit: Same as first input
  Selector : Selector  InputPortWidth=3  IndexOptions=Index vector (dialog)  Indices=[2 3 1]  OutputSizes=1
  Selector1 : Selector  InputPortWidth=3  IndexOptions=Index vector (dialog)  Indices=[3 1 2]  OutputSizes=1
  Selector2 : Selector  InputPortWidth=3  IndexOptions=Index vector (dialog)  Indices=[2 3 1]  OutputSizes=1
  Selector3 : Selector  InputPortWidth=3  IndexOptions=Index vector (dialog)  Indices=[3 1 2]  OutputSizes=1
  Sum : Sum  Inputs=+|-  SaturateOnIntegerOverflow=on  InputSameDT=on  OutDataTypeStr=Inherit: Same as first input
  c : Outport  InitialOutput=0
  wires:
  Selector3/1 -> Product1/1
  Selector2/1 -> Product1/2
  Product1/1 -> Sum/2
  Selector1/1 -> Product/2
  Product/1 -> Sum/1
  a/1 -> Selector3/1, Selector/1
  Selector/1 -> Product/1
  b/1 -> Selector2/1, Selector1/1
  Sum/1 -> c/1

== system TrajectoryTracking_2015b_000/Nonlinear Transformation/Position Error /Nonlinear Orientation Transformation ==
  theta : Inport
  SwitchSchedule : Inport  Port=2
  Demux : Demux  Outputs=3
  Display : Display
  Euler Angles to Angular Velocity Transfomration matrix : Subsystem
  Mux : Mux  Inputs=3
  Product : Product  Multiplication=Matrix(*)
  Transpose : Math  Operator=transpose  SaturateOnIntegerOverflow=on
  pitch_error : Subsystem
  roll_error : Subsystem
  yaw_error : Subsystem
  lambda_E : Outport
  wires:
  roll_error/1(roll_err) -> Mux/1
  yaw_error/1(yaw_err) -> Mux/3
  Demux/2 -> pitch_error/1(pitch)
  pitch_error/1(pitch_err) -> Mux/2
  Demux/3 -> yaw_error/1(yaw)
  theta/1 -> Euler Angles to Angular Velocity Transfomration matrix/1(theta), Demux/1
  Demux/1 -> roll_error/1(roll)
  Euler Angles to Angular Velocity Transfomration matrix/1(T) -> Transpose/1
  Transpose/1 -> Display/1, Product/1
  Mux/1 -> Product/2
  Product/1 -> lambda_E/1
  SwitchSchedule/1 -> yaw_error/2(SwitchSchedule), pitch_error/2(SwitchSchedule), roll_error/2(SwitchSchedule)

== system TrajectoryTracking_2015b_000/Nonlinear Transformation/Position Error /Nonlinear Position Transformation ==
  x,y,z : Inport
  theta : Inport  Port=2
  SwitchSchedule : Inport  Port=3
  Demux : Demux  Outputs=3
  Display : Display
  Euler Angles to inverse rotation matrix : Subsystem
  Mux : Mux  Inputs=3
  Product : Product  Multiplication=Matrix(*)
  x_error : Subsystem
  y_error : Subsystem
  z_error : Subsystem
  p_E : Outport
  wires:
  theta/1 -> Euler Angles to inverse rotation matrix/1(theta)
  Demux/3 -> z_error/1(z)
  Demux/2 -> y_error/1(y)
  Demux/1 -> x_error/1(x)
  x,y,z/1 -> Demux/1
  Product/1 -> p_E/1
  Mux/1 -> Product/2
  z_error/1(z_err) -> Mux/3
  x_error/1(x_err) -> Mux/1
  y_error/1(y_err) -> Mux/2
  Euler Angles to inverse rotation matrix/1(inv(R)) -> Display/1, Product/1
  SwitchSchedule/1 -> z_error/2(SwitchSchedule), y_error/2(SwitchSchedule), x_error/2(SwitchSchedule)

== system TrajectoryTracking_2015b_000/Nonlinear Transformation/Velocity Error /heave_error ==
  heave : Inport
  SwitchSchedule : Inport  Port=2
  Scope3 : Scope  NumInputPorts=2
  Sum5 : Sum  Inputs=|+-
  heave_d : Subsystem
  heave_err : Outport
  wires:
  heave/1 -> Scope3/1, Sum5/1
  Sum5/1 -> heave_err/1
  heave_d/1(heave_d) -> Scope3/2, Sum5/2
  SwitchSchedule/1 -> heave_d/1(SwitchSchedule)

== system TrajectoryTracking_2015b_000/Nonlinear Transformation/Velocity Error /pitch_error ==
  pitch : Inport
  SwitchSchedule : Inport  Port=2
  Scope3 : Scope  NumInputPorts=2
  Sum5 : Sum  Inputs=|+-
  pitch_d : Subsystem
  pitch_err : Outport
  wires:
  pitch/1 -> Scope3/1, Sum5/1
  Sum5/1 -> pitch_err/1
  SwitchSchedule/1 -> pitch_d/1(SwitchSchedule)
  pitch_d/1(pitch_d) -> Sum5/2, Scope3/2

== system TrajectoryTracking_2015b_000/Nonlinear Transformation/Velocity Error /roll_error ==
  roll : Inport
  SwitchSchedule : Inport  Port=2
  Scope3 : Scope  NumInputPorts=2
  Sum5 : Sum  Inputs=|+-
  roll_d : Subsystem
  roll_err : Outport
  wires:
  roll/1 -> Scope3/1, Sum5/1
  Sum5/1 -> roll_err/1
  SwitchSchedule/1 -> roll_d/1(SwitchSchedule)
  roll_d/1(roll_d) -> Scope3/2, Sum5/2

== system TrajectoryTracking_2015b_000/Nonlinear Transformation/Velocity Error /surge_error ==
  surge : Inport
  SwitchSchedule : Inport  Port=2
  Scope3 : Scope  NumInputPorts=2
  Sum5 : Sum  Inputs=|+-
  surge_d : Subsystem
  surge_err : Outport
  wires:
  surge/1 -> Scope3/1, Sum5/1
  Sum5/1 -> surge_err/1
  surge_d/1(surge_d) -> Scope3/2, Sum5/2
  SwitchSchedule/1 -> surge_d/1(SwitchSchedule)

== system TrajectoryTracking_2015b_000/Nonlinear Transformation/Velocity Error /sway_error ==
  sway : Inport
  SwitchSchedule : Inport  Port=2
  Scope3 : Scope  NumInputPorts=2
  Sum5 : Sum  Inputs=|+-
  sway_d : Subsystem
  sway_err : Outport
  wires:
  sway/1 -> Sum5/1
  Sum5/1 -> Scope3/1, sway_err/1
  SwitchSchedule/1 -> sway_d/1(SwitchSchedule)
  sway_d/1(sway_d) -> Scope3/2, Sum5/2

== system TrajectoryTracking_2015b_000/Nonlinear Transformation/Velocity Error /yaw_error ==
  pitch : Inport
  SwitchSchedule : Inport  Port=2
  Scope1 : Scope  NumInputPorts=2
  Scope3 : Scope  NumInputPorts=2
  Sum5 : Sum  Inputs=|+-
  yaw_d : Subsystem
  pitch_err : Outport
  wires:
  pitch/1 -> Scope1/1, Scope3/1, Sum5/1
  Sum5/1 -> pitch_err/1
  yaw_d/1(yaw_d) -> Sum5/2, Scope1/2, Scope3/2
  SwitchSchedule/1 -> yaw_d/1(SwitchSchedule)

== system TrajectoryTracking_2015b_000/Underwater Robot System/Underwater Robot System/DragCalculation ==
  nu : Inport
  Abs : Abs
  Constant : Constant  Value=veh.D
  Product : Product  Multiplication=Matrix(*)
  Product1 : Product
  HullDrag : Outport
  wires:
  Product/1 -> HullDrag/1
  Product1/1 -> Product/2
  Abs/1 -> Product1/1
  Constant/1 -> Product/1
  nu/1 -> Abs/1, Product1/2  "nu"

== system TrajectoryTracking_2015b_000/Underwater Robot System/Underwater Robot System/Dynamic2Kinematic(angular velocity) ==
  "p q r " : Inport
  Initial Integration Phi : Subsystem
  Initial Integration Value Generation Psi : Subsystem
  Initial Integration Value Generation Theta : Subsystem
  Mux1 : Mux  Inputs=3
  Rotation Angles to Direction Cosine Matrix : sharedtransform/Rotation Angles to Direction Cosine Matrix  rotationOrder=ZYX
      settings: SourceProductBaseCode=AE
  Selector : Selector  InputPortWidth=3  IndexOptions=Index vector (dialog)  Indices=[3 2 1]  OutputSizes=1
  phi theta psi : Integrator  InitialConditionSource=external
  phidot thetadot psidot : shared6dofsys/DCM & Euler Angles (Euler)/phidot thetadot psidot
  DCM : Outport
  Euler : Outport  Port=2
  Euler_dot : Outport  Port=3
  wires:
  Selector/1 -> Rotation Angles to Direction Cosine Matrix/1
  "p q r "/1 -> phidot thetadot psidot/1
  phi theta psi/1 -> phidot thetadot psidot/2, Selector/1, Euler/1
  phidot thetadot psidot/1 -> Euler_dot/1, phi theta psi/1
  Rotation Angles to Direction Cosine Matrix/1 -> DCM/1
  Initial Integration Value Generation Psi/1(Initial Orientation Integration Value) -> Mux1/3
  Initial Integration Value Generation Theta/1(Initial Theta Integration Value) -> Mux1/2
  Mux1/1 -> phi theta psi/2
  Initial Integration Phi/1(Initial Phi Integration Value) -> Mux1/1

== system TrajectoryTracking_2015b_000/Underwater Robot System/Underwater Robot System/Initial Integration Value Generation Generalised Location ==
  Constant : Constant  Value=0
  Mux : Mux  Inputs=3
  Initial Location Integration Value : Outport
  wires:
  Constant/1 -> Mux/1, Mux/3, Mux/2
  Mux/1 -> Initial Location Integration Value/1

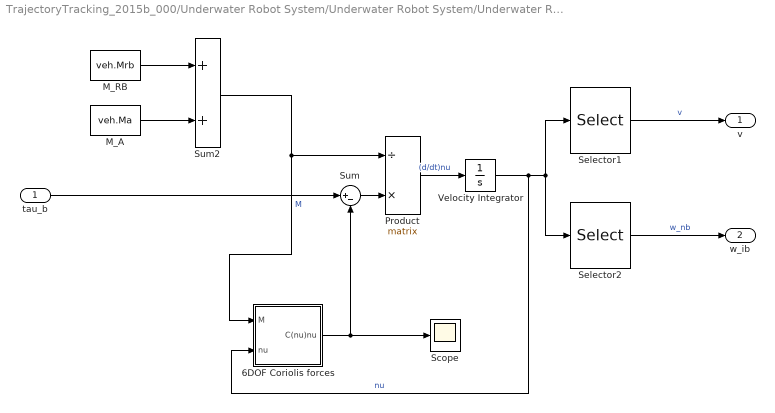
== system TrajectoryTracking_2015b_000/Underwater Robot System/Underwater Robot System/Underwater Robot Dynamics  ==
  tau_b : Inport
  6DOF Coriolis forces : Subsystem
  M_A : Constant  Value=veh.Ma
  M_RB : Constant  Value=veh.Mrb
  Product : Product  Inputs=/*  Multiplication=Matrix(*)  SaturateOnIntegerOverflow=on  OutDataTypeStr=Inherit: Same as first input
  Scope : Scope
  Selector1 : Selector  InputPortWidth=6  IndexOptions=Index vector (dialog)  Indices=[1 2 3]  OutputSizes=1
  Selector2 : Selector  InputPortWidth=6  IndexOptions=Index vector (dialog)  Indices=[4 5 6]  OutputSizes=1
  Sum : Sum  Inputs=|+-
  Sum2 : Sum  SaturateOnIntegerOverflow=on
  Velocity Integrator : Integrator
  v : Outport
  w_ib : Outport  Port=2
  wires:
  M_RB/1 -> Sum2/1
  M_A/1 -> Sum2/2
  Sum2/1 -> Product/1, 6DOF Coriolis forces/1(M)  "M"
  Selector2/1 -> w_ib/1  "w_nb"
  Product/1 -> Velocity Integrator/1  "(d/dt)nu"
  6DOF Coriolis forces/1(C(nu)nu) -> Sum/2, Scope/1
  Sum/1 -> Product/2
  Selector1/1 -> v/1  "v"
  Velocity Integrator/1 -> 6DOF Coriolis forces/2(nu), Selector2/1, Selector1/1  "nu"
  tau_b/1 -> Sum/1

== system TrajectoryTracking_2015b_000/Underwater Robot System/Underwater Robot System/transform to inertial world frame {i} ==
  v : Inport
  linear velocity transformation matrix : Inport  Port=2
  Product : Product  Multiplication=Matrix(*)  SaturateOnIntegerOverflow=on  InputSameDT=on  OutDataTypeStr=Inherit: Same as first input
  Reshape1 : Reshape  OutputDimensionality=Column vector (2-D)
  Reshape2 : Reshape
  Ve : Outport
  wires:
  Product/1 -> Reshape2/1
  Reshape1/1 -> Product/2
  v/1 -> Reshape1/1
  Reshape2/1 -> Ve/1
  linear velocity transformation matrix/1 -> Product/1

== system TrajectoryTracking_2015b_000/Actuator/Simplified Fin Model 1 /Drag Forces and Moments/Drag Force  ==
  AoA : Inport
  u : Inport  Port=2
  Constant : Constant  Value=0
  Gain1 : Gain  Gain=C_D*a_F*b_F
  Mux : Mux  Inputs=3
  Product : Product  Inputs=3
  q(V_ind) : Subsystem
  Drag Force : Outport
  wires:
  Mux/1 -> Drag Force/1
  Gain1/1 -> Product/1
  q(V_ind)/1(q(V_ind)) -> Gain1/1
  Product/1 -> Mux/1
  u/1 -> q(V_ind)/1(u)
  Constant/1 -> Mux/2, Mux/3
  AoA/1 -> Product/3, Product/2

== system TrajectoryTracking_2015b_000/Actuator/Simplified Fin Model 1 /Drag Forces and Moments/Geometric Center of fin ==
  Constant : Constant  Value=gama_F
  Gain : Gain  Gain=0.5*(d_H+a_F)
  Gain1 : Gain  Gain=0.5*(d_H+a_F)
  Mux : Mux  Inputs=3
  Trigonometric Function : Trigonometry  Operator=cos
  Trigonometric Function1 : Trigonometry
  x_F : Constant  Value=x_F
  r_F : Outport
  wires:
  x_F/1 -> Mux/1
  Constant/1 -> Trigonometric Function/1, Trigonometric Function1/1
  Mux/1 -> r_F/1
  Gain/1 -> Mux/2
  Trigonometric Function1/1 -> Gain/1
  Trigonometric Function/1 -> Gain1/1
  Gain1/1 -> Mux/3

== system TrajectoryTracking_2015b_000/Actuator/Simplified Fin Model 1 /Lift Forces and Moments/Geometric Center of fin ==
  Constant : Constant  Value=gama_F
  Gain : Gain  Gain=0.5*(d_H+a_F)
  Gain1 : Gain  Gain=0.5*(d_H+a_F)
  Mux : Mux  Inputs=3
  Trigonometric Function : Trigonometry  Operator=cos
  Trigonometric Function1 : Trigonometry
  x_F : Constant  Value=x_F
  r_F : Outport
  wires:
  x_F/1 -> Mux/1
  Constant/1 -> Trigonometric Function/1, Trigonometric Function1/1
  Mux/1 -> r_F/1
  Gain/1 -> Mux/2
  Trigonometric Function1/1 -> Gain/1
  Trigonometric Function/1 -> Gain1/1
  Gain1/1 -> Mux/3

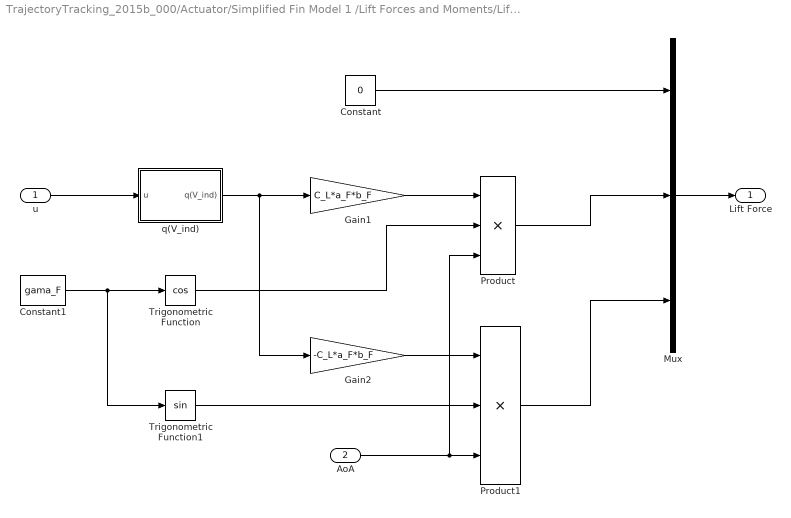
== system TrajectoryTracking_2015b_000/Actuator/Simplified Fin Model 1 /Lift Forces and Moments/Lift Force  ==
  u : Inport
  AoA : Inport  Port=2
  Constant : Constant  Value=0
  Constant1 : Constant  Value=gama_F
  Gain1 : Gain  Gain=C_L*a_F*b_F
  Gain2 : Gain  Gain=-C_L*a_F*b_F
  Mux : Mux  Inputs=3
  Product : Product  Inputs=3
  Product1 : Product  Inputs=3
  Trigonometric Function : Trigonometry  Operator=cos
  Trigonometric Function1 : Trigonometry
  q(V_ind) : Subsystem
  Lift Force : Outport
  wires:
  u/1 -> q(V_ind)/1(u)
  q(V_ind)/1(q(V_ind)) -> Gain2/1, Gain1/1
  Gain1/1 -> Product/1
  Trigonometric Function/1 -> Product/2
  Mux/1 -> Lift Force/1
  Gain2/1 -> Product1/1
  Trigonometric Function1/1 -> Product1/2
  Constant/1 -> Mux/1
  Product/1 -> Mux/2
  Product1/1 -> Mux/3
  AoA/1 -> Product/3, Product1/3
  Constant1/1 -> Trigonometric Function1/1, Trigonometric Function/1

== system TrajectoryTracking_2015b_000/Actuator/Simplified Fin Model 2/Drag Forces and Moments/Drag Force  ==
  AoA : Inport
  u : Inport  Port=2
  Constant : Constant  Value=0
  Gain1 : Gain  Gain=C_D*a_F*b_F
  Mux : Mux  Inputs=3
  Product : Product  Inputs=3
  q(V_ind) : Subsystem
  Drag Force : Outport
  wires:
  Mux/1 -> Drag Force/1
  Gain1/1 -> Product/1
  q(V_ind)/1(q(V_ind)) -> Gain1/1
  Product/1 -> Mux/1
  u/1 -> q(V_ind)/1(u)
  Constant/1 -> Mux/2, Mux/3
  AoA/1 -> Product/3, Product/2

== system TrajectoryTracking_2015b_000/Actuator/Simplified Fin Model 2/Drag Forces and Moments/Geometric Center of fin ==
  Constant : Constant  Value=gama_F
  Gain : Gain  Gain=0.5*(d_H+a_F)
  Gain1 : Gain  Gain=0.5*(d_H+a_F)
  Mux : Mux  Inputs=3
  Trigonometric Function : Trigonometry  Operator=cos
  Trigonometric Function1 : Trigonometry
  x_F : Constant  Value=x_F
  r_F : Outport
  wires:
  x_F/1 -> Mux/1
  Constant/1 -> Trigonometric Function/1, Trigonometric Function1/1
  Mux/1 -> r_F/1
  Gain/1 -> Mux/2
  Trigonometric Function1/1 -> Gain/1
  Trigonometric Function/1 -> Gain1/1
  Gain1/1 -> Mux/3

== system TrajectoryTracking_2015b_000/Actuator/Simplified Fin Model 2/Lift Forces and Moments/Geometric Center of fin ==
  Constant : Constant  Value=gama_F
  Gain : Gain  Gain=0.5*(d_H+a_F)
  Gain1 : Gain  Gain=0.5*(d_H+a_F)
  Mux : Mux  Inputs=3
  Trigonometric Function : Trigonometry  Operator=cos
  Trigonometric Function1 : Trigonometry
  x_F : Constant  Value=x_F
  r_F : Outport
  wires:
  x_F/1 -> Mux/1
  Constant/1 -> Trigonometric Function/1, Trigonometric Function1/1
  Mux/1 -> r_F/1
  Gain/1 -> Mux/2
  Trigonometric Function1/1 -> Gain/1
  Trigonometric Function/1 -> Gain1/1
  Gain1/1 -> Mux/3

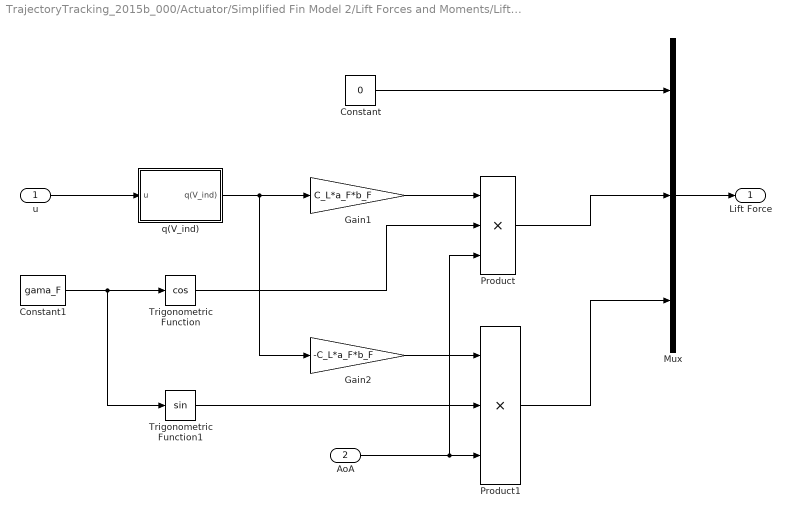
== system TrajectoryTracking_2015b_000/Actuator/Simplified Fin Model 2/Lift Forces and Moments/Lift Force  ==
  u : Inport
  AoA : Inport  Port=2
  Constant : Constant  Value=0
  Constant1 : Constant  Value=gama_F
  Gain1 : Gain  Gain=C_L*a_F*b_F
  Gain2 : Gain  Gain=-C_L*a_F*b_F
  Mux : Mux  Inputs=3
  Product : Product  Inputs=3
  Product1 : Product  Inputs=3
  Trigonometric Function : Trigonometry  Operator=cos
  Trigonometric Function1 : Trigonometry
  q(V_ind) : Subsystem
  Lift Force : Outport
  wires:
  u/1 -> q(V_ind)/1(u)
  q(V_ind)/1(q(V_ind)) -> Gain2/1, Gain1/1
  Gain1/1 -> Product/1
  Trigonometric Function/1 -> Product/2
  Mux/1 -> Lift Force/1
  Gain2/1 -> Product1/1
  Trigonometric Function1/1 -> Product1/2
  Constant/1 -> Mux/1
  Product/1 -> Mux/2
  Product1/1 -> Mux/3
  AoA/1 -> Product/3, Product1/3
  Constant1/1 -> Trigonometric Function1/1, Trigonometric Function/1

== system TrajectoryTracking_2015b_000/Actuator/Simplified Fin Model 3/Drag Forces and Moments/Drag Force  ==
  AoA : Inport
  u : Inport  Port=2
  Constant : Constant  Value=0
  Gain1 : Gain  Gain=C_D*a_F*b_F
  Mux : Mux  Inputs=3
  Product : Product  Inputs=3
  q(V_ind) : Subsystem
  Drag Force : Outport
  wires:
  Mux/1 -> Drag Force/1
  Gain1/1 -> Product/1
  q(V_ind)/1(q(V_ind)) -> Gain1/1
  Product/1 -> Mux/1
  u/1 -> q(V_ind)/1(u)
  Constant/1 -> Mux/2, Mux/3
  AoA/1 -> Product/3, Product/2

== system TrajectoryTracking_2015b_000/Actuator/Simplified Fin Model 3/Drag Forces and Moments/Geometric Center of fin ==
  Constant : Constant  Value=gama_F
  Gain : Gain  Gain=0.5*(d_H+a_F)
  Gain1 : Gain  Gain=0.5*(d_H+a_F)
  Mux : Mux  Inputs=3
  Trigonometric Function : Trigonometry  Operator=cos
  Trigonometric Function1 : Trigonometry
  x_F : Constant  Value=x_F
  r_F : Outport
  wires:
  x_F/1 -> Mux/1
  Constant/1 -> Trigonometric Function/1, Trigonometric Function1/1
  Mux/1 -> r_F/1
  Gain/1 -> Mux/2
  Trigonometric Function1/1 -> Gain/1
  Trigonometric Function/1 -> Gain1/1
  Gain1/1 -> Mux/3

== system TrajectoryTracking_2015b_000/Actuator/Simplified Fin Model 3/Lift Forces and Moments/Geometric Center of fin ==
  Constant : Constant  Value=gama_F
  Gain : Gain  Gain=0.5*(d_H+a_F)
  Gain1 : Gain  Gain=0.5*(d_H+a_F)
  Mux : Mux  Inputs=3
  Trigonometric Function : Trigonometry  Operator=cos
  Trigonometric Function1 : Trigonometry
  x_F : Constant  Value=x_F
  r_F : Outport
  wires:
  x_F/1 -> Mux/1
  Constant/1 -> Trigonometric Function/1, Trigonometric Function1/1
  Mux/1 -> r_F/1
  Gain/1 -> Mux/2
  Trigonometric Function1/1 -> Gain/1
  Trigonometric Function/1 -> Gain1/1
  Gain1/1 -> Mux/3

== system TrajectoryTracking_2015b_000/Actuator/Simplified Fin Model 3/Lift Forces and Moments/Lift Force  ==
  u : Inport
  AoA : Inport  Port=2
  Constant : Constant  Value=0
  Constant1 : Constant  Value=gama_F
  Gain1 : Gain  Gain=C_L*a_F*b_F
  Gain2 : Gain  Gain=-C_L*a_F*b_F
  Mux : Mux  Inputs=3
  Product : Product  Inputs=3
  Product1 : Product  Inputs=3
  Trigonometric Function : Trigonometry  Operator=cos
  Trigonometric Function1 : Trigonometry
  q(V_ind) : Subsystem
  Lift Force : Outport
  wires:
  u/1 -> q(V_ind)/1(u)
  q(V_ind)/1(q(V_ind)) -> Gain2/1, Gain1/1
  Gain1/1 -> Product/1
  Trigonometric Function/1 -> Product/2
  Mux/1 -> Lift Force/1
  Gain2/1 -> Product1/1
  Trigonometric Function1/1 -> Product1/2
  Constant/1 -> Mux/1
  Product/1 -> Mux/2
  Product1/1 -> Mux/3
  AoA/1 -> Product/3, Product1/3
  Constant1/1 -> Trigonometric Function1/1, Trigonometric Function/1

== system TrajectoryTracking_2015b_000/Actuator/Simplified Fin Model 4/Drag Forces and Moments/Drag Force  ==
  AoA : Inport
  u : Inport  Port=2
  Constant : Constant  Value=0
  Gain1 : Gain  Gain=C_D*a_F*b_F
  Mux : Mux  Inputs=3
  Product : Product  Inputs=3
  q(V_ind) : Subsystem
  Drag Force : Outport
  wires:
  Mux/1 -> Drag Force/1
  Gain1/1 -> Product/1
  q(V_ind)/1(q(V_ind)) -> Gain1/1
  Product/1 -> Mux/1
  u/1 -> q(V_ind)/1(u)
  Constant/1 -> Mux/2, Mux/3
  AoA/1 -> Product/3, Product/2

== system TrajectoryTracking_2015b_000/Actuator/Simplified Fin Model 4/Drag Forces and Moments/Geometric Center of fin ==
  Constant : Constant  Value=gama_F
  Gain : Gain  Gain=0.5*(d_H+a_F)
  Gain1 : Gain  Gain=0.5*(d_H+a_F)
  Mux : Mux  Inputs=3
  Trigonometric Function : Trigonometry  Operator=cos
  Trigonometric Function1 : Trigonometry
  x_F : Constant  Value=x_F
  r_F : Outport
  wires:
  x_F/1 -> Mux/1
  Constant/1 -> Trigonometric Function/1, Trigonometric Function1/1
  Mux/1 -> r_F/1
  Gain/1 -> Mux/2
  Trigonometric Function1/1 -> Gain/1
  Trigonometric Function/1 -> Gain1/1
  Gain1/1 -> Mux/3

== system TrajectoryTracking_2015b_000/Actuator/Simplified Fin Model 4/Lift Forces and Moments/Geometric Center of fin ==
  Constant : Constant  Value=gama_F
  Gain : Gain  Gain=0.5*(d_H+a_F)
  Gain1 : Gain  Gain=0.5*(d_H+a_F)
  Mux : Mux  Inputs=3
  Trigonometric Function : Trigonometry  Operator=cos
  Trigonometric Function1 : Trigonometry
  x_F : Constant  Value=x_F
  r_F : Outport
  wires:
  x_F/1 -> Mux/1
  Constant/1 -> Trigonometric Function/1, Trigonometric Function1/1
  Mux/1 -> r_F/1
  Gain/1 -> Mux/2
  Trigonometric Function1/1 -> Gain/1
  Trigonometric Function/1 -> Gain1/1
  Gain1/1 -> Mux/3

== system TrajectoryTracking_2015b_000/Actuator/Simplified Fin Model 4/Lift Forces and Moments/Lift Force  ==
  u : Inport
  AoA : Inport  Port=2
  Constant : Constant  Value=0
  Constant1 : Constant  Value=gama_F
  Gain1 : Gain  Gain=C_L*a_F*b_F
  Gain2 : Gain  Gain=-C_L*a_F*b_F
  Mux : Mux  Inputs=3
  Product : Product  Inputs=3
  Product1 : Product  Inputs=3
  Trigonometric Function : Trigonometry  Operator=cos
  Trigonometric Function1 : Trigonometry
  q(V_ind) : Subsystem
  Lift Force : Outport
  wires:
  u/1 -> q(V_ind)/1(u)
  q(V_ind)/1(q(V_ind)) -> Gain2/1, Gain1/1
  Gain1/1 -> Product/1
  Trigonometric Function/1 -> Product/2
  Mux/1 -> Lift Force/1
  Gain2/1 -> Product1/1
  Trigonometric Function1/1 -> Product1/2
  Constant/1 -> Mux/1
  Product/1 -> Mux/2
  Product1/1 -> Mux/3
  AoA/1 -> Product/3, Product1/3
  Constant1/1 -> Trigonometric Function1/1, Trigonometric Function/1
